simulink model "Interprete_DTFT_Spectrum1"  (R2014a)
settings: Solver=FixedStepDiscrete  StartTime=0.0  StopTime=6e-3  FixedStep=Ts/10  RelTol=1e-3
PreLoadFcn:
  | close all
InitFcn:
  | clear all
  | clc
  | 
  | ms=1e-3;
  | KHz=1e3;
  | 
  | Ts=0.01*ms;
  | Fs=1/Ts;
  | 
  | %If not previously done create figures for DTFT plots
  | if ~ishandle(1)
  |      figure(1)
  |      set(1,'Position', [150 550 500 350]);
  | end
  | if ~ishandle(2)
  |     figure(2)
  |     set(2,'Position', [150 110 500 350]);
  | end
StopFcn:
  | n=[0:length(simout)-1];
  | w=[-500:500]*pi/500;
  | X=dtft(simout,n,w);
  | magX=abs(X);
  | %magX=magX/max(magX);
  | TotalTime=tout(end);
  | N=TotalTime*Fs;
  | magX=magX/N;
  | 
  | figure(1)
  | plot((w/pi),magX,'LineWidth',2)
  | grid on
  | set(gca,'ylim',[0 2],'Xtick',[-1:.2: 1])
  | xlabel(' \omega/\pi, Nyquist Normalized Frequency (Samples per Half Cycle)');
  | ylabel('magntidue(dtft)')
  | 
  | figure(2)
  | plot(w*Fs/(2*pi*KHz),magX,'LineWidth',2)
  | grid on
  | set(gca,'ylim',[0 2],'Xtick',[-50:10: 50])
  | xlabel('Physical Frequency,\Omega, (KHz)')
undefined symbols (not defined in the file or in its folder): j
CloseFcn:
  | close all
settings Model: Creator=Alfred  LastModifiedBy=Edwards
settings DataIOCC: SignalLoggingSaveFormat=ModelDataLogs
settings OptimizationCC: ExpressionDepthLimit=2147483647
settings DebuggingCC: UnderspecifiedInitializationDetection=Classic  MultiTaskRateTransMsg=warning  FcnCallInpInsideContextMsg=UseLocalSettings  StateNameClashWarn=warning
settings GRTTargetCC: CombineOutputUpdateFcns=off  GRTInterface=on

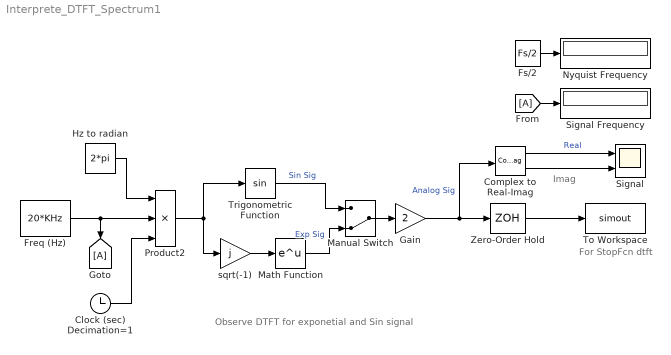
== system Interprete_DTFT_Spectrum1 ==
  note: Observe DTFT for exponetial and Sin signal
  note: Imag
  note: For StopFcn dtft
  " Signal" : Scope  NumInputPorts=2
      settings: TimeRange=0.0006  YMin=-4~-4  YMax=4~4
  Clock (sec) Decimation=1 : Clock
  Complex to Real-Imag : ComplexToRealImag
  Freq (Hz) : Constant  Value=20*KHz
  Fs/2 : Constant  Value=Fs/2
  Gain : Gain  Gain=2
  "Hz to radian " : Constant  Value=2*pi
  Manual Switch : ManualSwitch  CurrentSetting=0
  Math Function : Math  SaturateOnIntegerOverflow=on
  Nyquist Frequency : Display
  Product2 : Product  Inputs=3  RndMeth=Zero
  Signal Frequency : Display
  To Workspace : ToWorkspace  VariableName=simout  SampleTime=-1
  Trigonometric Function : Trigonometry  OutputSignalType=complex
  Zero-Order Hold : ZeroOrderHold  SampleTime=Ts
  sqrt(-1) : Gain  Gain=j
  wires:
  Freq (Hz)/1 -> [A], Product2/2
  Clock (sec) Decimation=1/1 -> Product2/3
  "Hz to radian "/1 -> Product2/1
  Product2/1 -> sqrt(-1)/1, Trigonometric Function/1
  [A] -> Signal Frequency/1
  Fs/2/1 -> Nyquist Frequency/1
  sqrt(-1)/1 -> Math Function/1
  Gain/1 -> Complex to Real-Imag/1, Zero-Order Hold/1  "Analog Sig"
  Zero-Order Hold/1 -> To Workspace/1
  Math Function/1 -> Manual Switch/2  "Exp Sig"
  Manual Switch/1 -> Gain/1
  Trigonometric Function/1 -> Manual Switch/1  "Sin Sig"
  Complex to Real-Imag/2 -> " Signal"/2
  Complex to Real-Imag/1 -> " Signal"/1  "Real"
